simulink model "Hilbert_Curve_Trajectory_Generator"  (R2023a)
settings: Solver=ode4  StartTime=0.0  StopTime=Tend  FixedStep=Ts  RelTol=1e-3
values from neighbouring files (symbols this model uses):
  alpha = 2    [trajectory_csv_generator.m]
undefined symbols (not defined in the file or in its folder): sigbuilder_block
settings Model: Creator=PhDstudent1  LastModifiedBy=Juan Augusto Paredes
settings ModelReferenceCC: EnableRefExpFcnMdlSchedulingChecks=on

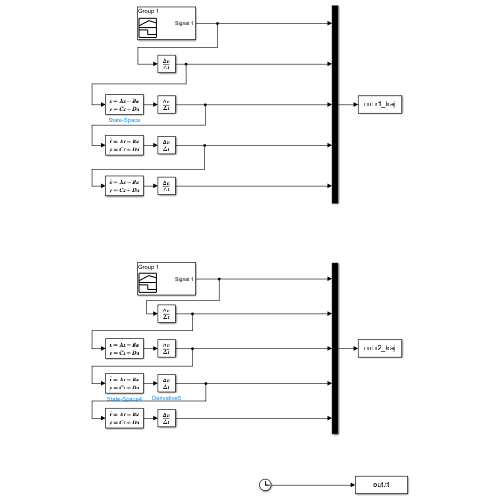
[thumbnail: Simulink's stored preview of the top-level diagram]
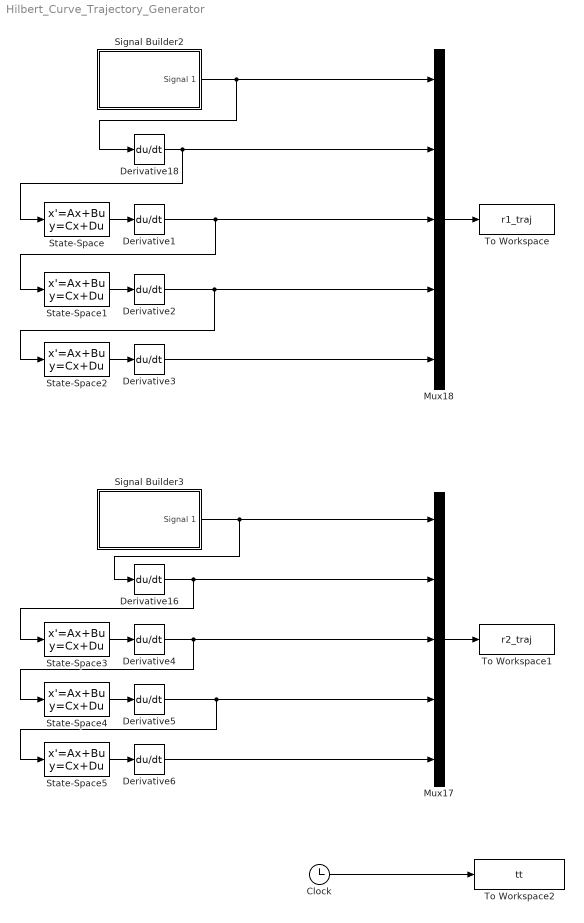
== system Hilbert_Curve_Trajectory_Generator ==
  Clock : Clock
  Derivative{1..6,16,18} (8 alike) : Derivative
  Mux17 : Mux  Inputs=5
  Mux18 : Mux  Inputs=5
  Signal Builder2 : Subsystem  Tag=STV Subsys  LoadFcn=sigbuilder_block('load');  StartFcn=sigbuilder_block('start');  StopFcn=sigbuilder_block('stop');  ClipboardFcn=sigbuilder_block('clipboard');  mask(Sigbuilder block){tuvar=[0:10]}
      mask help: Simulink:masks:SigbuilderBlock_MD
      mask init:
      | if ~strcmp(get_param(bdroot(gcbh),'SimulationStatus'),'stopped') tuvar = sigbuilder_block('maskInit'); end
      settings: CopyFcn=sigbuilder_block('copy');  DeleteFcn=sigbuilder_block('delete');  ModelCloseFcn=sigbuilder_block('modelClose');  PreSaveFcn=sigbuilder_block('preSave');  PauseFcn=sigbuilder_block('pause');  ContinueFcn=sigbuilder_block('continue');  NameChangeFcn=sigbuilder_block('namechange');  OpenFcn=sigbuilder_block('open',[438.6 146.4 550.8 400.2 ]);  CloseFcn=sigbuilder_block('close');
      mask Display: plot(0, 0, 100, 100,[2, 2, 32, 32, 2], [68, 8, 8, 68, 68],[32, 2], [38, 38], [32, 19, 2],[53, 60, 44], [32, 17, 17, 2],[16, 16, 31, 31]);txt = getActiveGroup(gcbh);text(2, 100, txt,'verticalAlignment', 'top');
  Signal Builder3 : Subsystem  Tag=STV Subsys  LoadFcn=sigbuilder_block('load');  StartFcn=sigbuilder_block('start');  StopFcn=sigbuilder_block('stop');  ClipboardFcn=sigbuilder_block('clipboard');  mask(Sigbuilder block){tuvar=[0:10]}
      mask help: Simulink:masks:SigbuilderBlock_MD
      mask init:
      | if ~strcmp(get_param(bdroot(gcbh),'SimulationStatus'),'stopped') tuvar = sigbuilder_block('maskInit'); end
      settings: CopyFcn=sigbuilder_block('copy');  DeleteFcn=sigbuilder_block('delete');  ModelCloseFcn=sigbuilder_block('modelClose');  PreSaveFcn=sigbuilder_block('preSave');  PauseFcn=sigbuilder_block('pause');  ContinueFcn=sigbuilder_block('continue');  NameChangeFcn=sigbuilder_block('namechange');  OpenFcn=sigbuilder_block('open',[437.6 199.2 550.4 400 ]);  CloseFcn=sigbuilder_block('close');
      mask Display: plot(0, 0, 100, 100,[2, 2, 32, 32, 2], [68, 8, 8, 68, 68],[32, 2], [38, 38], [32, 19, 2],[53, 60, 44], [32, 17, 17, 2],[16, 16, 31, 31]);txt = getActiveGroup(gcbh);text(2, 100, txt,'verticalAlignment', 'top');
  State-Space{,1..5} (6 alike) : StateSpace  A=-alpha  B=alpha  D=0  InitialCondition=0
  To Workspace : ToWorkspace  VariableName=r1_traj  SampleTime=-1
  To Workspace1 : ToWorkspace  VariableName=r2_traj  SampleTime=-1
  To Workspace2 : ToWorkspace  VariableName=tt  SampleTime=-1
  wires:
  State-Space3/1 -> Derivative4/1
  State-Space2/1 -> Derivative3/1
  State-Space1/1 -> Derivative2/1
  State-Space/1 -> Derivative1/1
  Derivative18/1 -> State-Space/1, Mux18/2
  Derivative6/1 -> Mux17/5
  Derivative5/1 -> State-Space5/1, Mux17/4
  Derivative4/1 -> State-Space4/1, Mux17/3
  Derivative3/1 -> Mux18/5
  Derivative2/1 -> State-Space2/1, Mux18/4
  Derivative1/1 -> State-Space1/1, Mux18/3
  Signal Builder3/1(Signal 1) -> Derivative16/1, Mux17/1
  Derivative16/1 -> State-Space3/1, Mux17/2
  Signal Builder2/1(Signal 1) -> Derivative18/1, Mux18/1
  State-Space4/1 -> Derivative5/1
  State-Space5/1 -> Derivative6/1
  Clock/1 -> To Workspace2/1
  Mux18/1 -> To Workspace/1
  Mux17/1 -> To Workspace1/1

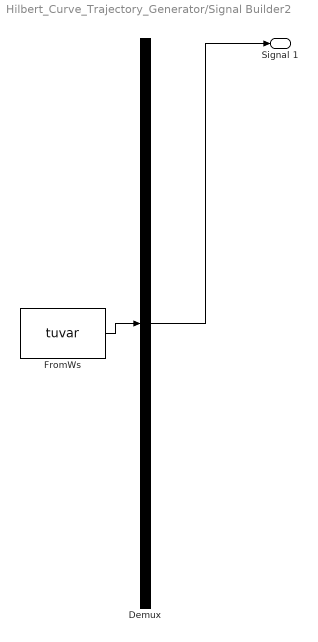
== system Hilbert_Curve_Trajectory_Generator/Signal Builder2 ==
  Demux : Demux  Tag=STV Demux  Outputs=1
      settings: DisplayOption=none
  FromWs : FromWorkspace  Tag=STV FromWs  VariableName=tuvar
      SigBuilderData=|
      | common.afterFinalStr = 'Extrapolate'
      | common.sampleTime = 0
      | dataSet.timeRange = [0 110]
      | dataSet.name = 'Group 1'
      | sbobj.Groups.Name = 'Group 1'
      | sbobj.Groups.Signals.Name = 'Signal 1'
      | sbobj.Groups.Signals.XData = [0 7 14 21 35 42 49 56 65 70 84 91 98 105 110]
      | sbobj.Groups.Signals.YData = [0 4 4 0 0 4 4 8 8 12 12 8 8 12 12]
      | sbobj.Groups.TimeRange = [0 110]
  Signal 1 : Outport  Tag=STV Outport
  wires:
  Demux/1 -> Signal 1/1
  FromWs/1 -> Demux/1

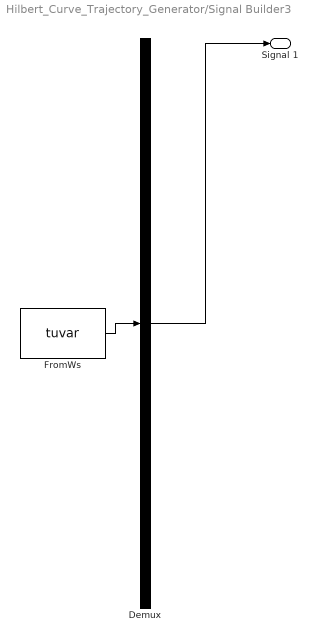
== system Hilbert_Curve_Trajectory_Generator/Signal Builder3 ==
  Demux : Demux  Tag=STV Demux  Outputs=1
      settings: DisplayOption=none
  FromWs : FromWorkspace  Tag=STV FromWs  VariableName=tuvar
      SigBuilderData=|
      | common.afterFinalStr = 'Extrapolate'
      | common.sampleTime = 0
      | dataSet.timeRange = [0 110]
      | dataSet.name = 'Group 1'
      | sbobj.Groups.Name = 'Group 1'
      | sbobj.Groups.Signals.Name = 'Signal 1'
      | sbobj.Groups.Signals.XData = [0 7 14 21 35 42 49 56 63 70 84 91 98 105 110]
      | sbobj.Groups.Signals.YData = [0 0 -7 -7 -21 -21 -14 -14 -21 -21 -7 -7 0 0 0]
      | sbobj.Groups.TimeRange = [0 110]
  Signal 1 : Outport  Tag=STV Outport
  wires:
  Demux/1 -> Signal 1/1
  FromWs/1 -> Demux/1
